simulink model "course_loop"  (R2016b)
settings: Solver=ode45  StartTime=0.0  StopTime=100  RelTol=1e-3  EnableMultiTasking=on
InitFcn:
  | param_chap6
values from neighbouring files (symbols this model uses):
  P = (eye(2,2) -L*C)*P    [estimate_states.m]
undefined symbols (not defined in the file or in its folder): phi_max
settings Model: Creator=beard  LastModifiedBy=Chui Vanfleet
settings DataIOCC: LimitDataPoints=on  SaveFormat=Array  SignalLoggingSaveFormat=ModelDataLogs
settings OptimizationCC: ExpressionDepthLimit=2147483647  LifeSpan=inf
settings DebuggingCC: UnderspecifiedInitializationDetection=Classic  MergeDetectMultiDrivingBlocksExec=none  SolverPrmCheckMsg=warning  FcnCallInpInsideContextMsg=warning  StateNameClashWarn=warning  SFUnexpectedBacktrackingDiag=warning  SFNoUnconditionalDefaultTransitionDiag=warning  SFExecutionAtInitializationDiag=none
settings HardwareCC: ProdBitPerPointer=32  ProdBitPerSizeT=32  ProdBitPerPtrDiffT=32  ProdLargestAtomicFloat=None  ProdIntDivRoundTo=Undefined  ProdEndianess=Unspecified  ProdWordSize=32  ProdHWDeviceType=32-bit Generic
settings ModelReferenceCC: PropagateSignalLabelsOutOfModel=off
settings GRTTargetCC: TargetLangStandard=C89/C90 (ANSI)  GeneratePreprocessorConditionals=Disable all  CombineOutputUpdateFcns=off  GRTInterface=on
settings ConfigComp: CovMetricSettings=dw  CovHtmlReporting=on  CovSaveCumulativeToWorkspaceVar=on  CovSaveSingleToWorkspaceVar=on  CovExternalEMLEnable=off  CovSFcnEnable=off

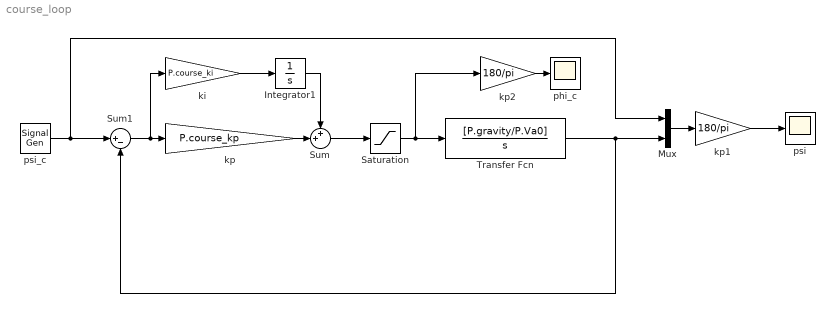
== system course_loop ==
  Integrator1 : Integrator
  Mux : Mux  Inputs=2
  Saturation : Saturate  UpperLimit=phi_max  LowerLimit=-phi_max
  Sum : Sum  Inputs=++|
  Sum1 : Sum  Inputs=|+-
  Transfer Fcn : TransferFcn  Numerator=[P.gravity/P.Va0]  Denominator=[1 0]
  ki : Gain  Gain=P.course_ki
  kp : Gain  Gain=P.course_kp
  kp1 : Gain  Gain=180/pi
  kp2 : Gain  Gain=180/pi
  phi_c : Scope
  psi : Scope
  psi_c : SignalGenerator  WaveForm=square  Amplitude=25*pi/180  Frequency=.02
  wires:
  Transfer Fcn/1 -> Sum1/2, Mux/2
  Saturation/1 -> Transfer Fcn/1, kp2/1
  Sum/1 -> Saturation/1
  kp/1 -> Sum/2
  Sum1/1 -> kp/1, ki/1
  ki/1 -> Integrator1/1
  Integrator1/1 -> Sum/1
  psi_c/1 -> Sum1/1, Mux/1
  kp1/1 -> psi/1
  Mux/1 -> kp1/1
  kp2/1 -> phi_c/1
